simulink model "Vehicle_Model"  (R2018b)
settings: Solver=VariableStepAuto  StartTime=0.0  StopTime=60  FixedStep=0.00000000000000000000000000000000000000001  RelTol=1e-3
undefined symbols (not defined in the file or in its folder): Chassis8_Initial, Initial
(part 2 of 3)

== matlab function Vehicle_Model/MATLAB Function ==
  data: Z output; z input; m_C input; m_WFR input; m_WFL input; m_WRR input; m_WRL input; I_Cy input; I_CFx input; I_CRx input; a input; b input; d_F input; e_F input; d_R input; e_R input; k_SFR input; k_SFL input; k_SRR input; k_SRL input; k_TFR input; k_TFL input; k_TRR input; k_TRL input; c_SFR input; c_SFL input; c_SRR input; c_SRL input; c_TFR input; c_TFL input; c_TRR input; c_TRL input; k_C input; c_C input; F_z input; M_y input; M_xF input; M_xR input; y_FR input; y_FL input; y_RR input; y_RL input; ydot_FR input; ydot_FL input; ydot_RR input; ydot_RL input
function Z = Chassis8(z,m_C,m_WFR,m_WFL,m_WRR,m_WRL,...
    I_Cy,I_CFx,I_CRx,a,b,d_F,e_F,d_R,e_R,k_SFR,k_SFL,k_SRR,k_SRL,...
    k_TFR,k_TFL,k_TRR,k_TRL,c_SFR,c_SFL,c_SRR,c_SRL,c_TFR,c_TFL,...
    c_TRR,c_TRL,k_C,c_C,F_z,M_y,M_xF,M_xR,y_FR,y_FL,y_RR,y_RL,...
    ydot_FR,ydot_FL,ydot_RR,ydot_RL)

Z = [z(2);...
    ...
    (1/m_C) * (F_z...
    + k_SRR * (z(9) - z(1) - b * z(3) + e_R * z(7))...
    + k_SFR * (z(11) - z(1) + a * z(3) + e_F * z(5))...
    + k_SFL * (z(13) - z(1) + a * z(3) - d_F * z(5))...
    + k_SRL * (z(15) - z(1) - b * z(3) - d_R * z(7))...
    + c_SRR * (z(10) - z(2) - b * z(4) + e_R * z(8))...
    + c_SFR * (z(12) - z(2) + a * z(4) + e_F * z(6))...
    + c_SFL * (z(14) - z(2) + a * z(4) - d_F * z(6))...
    + c_SRL * (z(16) - z(2) - b * z(4) - d_R * z(8)));...
    ...
    z(4);...
    ...
    (1/I_Cy) * (M_y...
    + b * k_SRR * (z(9) - z(1) - b * z(3) + e_R * z(7))...
    - a * k_SFR * (z(11) - z(1) + a * z(3) + e_F * z(5))...
    - a * k_SFL * (z(13) - z(1) + a * z(3) - d_F * z(5))...
    + b * k_SRL * (z(15) - z(1) - b * z(3) - d_R * z(7))...
    + b * c_SRR * (z(10) - z(2) - b * z(4) + e_R * z(8))...
    - a * c_SFR * (z(12) - z(2) + a * z(4) + e_F * z(6))...
    - a * c_SFL * (z(14) - z(2) + a * z(4) - d_F * z(6))...
    + b * c_SRL * (z(16) - z(2) - b * z(4) - d_R * z(8)));...
    ...
    z(6);...
    ...
    (1/I_CFx) * (M_xF...
    - e_F * k_SFR * (z(11) - z(1) + a * z(3) + e_F * z(5))...
    + d_F * k_SFL * (z(13) - z(1) + a * z(3) - d_F * z(5))...
    - k_C * (z(5) - z(7))...
    - e_F * c_SFR * (z(12) - z(2) + a * z(4) + e_F * z(6))...
    + d_F * c_SFL * (z(14) - z(2) + a * z(4) - d_F * z(6))...
    - c_C * (z(6) - z(8)));...
    ...
    z(8);...
    ...
    (1/I_CRx) * (M_xR...
    - e_R * k_SRR * (z(9) - z(1) - b * z(3) + e_R * z(7))...
    + d_F * k_SRL * (z(15) - z(1) - b * z(3) - d_R * z(7))...
    + k_C * (z(5) - z(7))...
    - e_R * c_SRR * (z(10) - z(2) - b * z(4) + e_R * z(8))...
    + d_F * c_SRL * (z(16) - z(2) - b * z(4) - d_R * z(8))...
    + c_C * (z(6) - z(8)));...
    ...
    z(10);...
    ...
    (1/m_WRR) * (0 ...
    + k_TRR * (y_RR - z(9))...
    - k_SRR * (z(9) - z(1) - b * z(3) + e_R * z(7))...
    + c_TRR * (ydot_RR - z(10))...
    - c_SRR * (z(10) - z(2) - b * z(4) + e_R * z(8)));...
    ...
    z(12);...
    ...
    (1/m_WFR) * (0 ...
    + k_TFR * (y_FR - z(11))...
    - k_SFR * (z(11) - z(1) + a * z(3) + e_F * z(5))...
    + c_TFR * (ydot_FR - z(12))...
    - c_SFR * (z(12) - z(2) + a * z(4) + e_F * z(6)));...
    ...
    z(14);...
    ...
    (1/m_WFL) * (0 ...
    + k_TFL * (y_FL - z(13))...
    - k_SFL * (z(13) - z(1) + a * z(3) - d_F * z(5))...
    + c_TFL * (ydot_FL - z(14))...
    - c_SFL * (z(14) - z(2) + a * z(4) - d_F * z(6)));...
    ...
    z(16);...
    ...
    (1/m_WRL) * (0 ...
    + k_TRL * (y_RL - z(15))...
    - k_SRL * (z(15) - z(1) - b * z(3) - d_R * z(7))...
    + c_TRL * (ydot_RL - z(16))...
    - c_SRL * (z(16) - z(2) - b * z(4) - d_R * z(8)))...
    ];

end

== matlab function Vehicle_Model/MATLAB Function2 ==
  data: F_z output; M_y output; M_xF output; M_xR output
function [F_z,M_y,M_xF,M_xR] = Forces

% Forces & Moments
g = 9.81;
F_z = -500; %-m_C * g;
M_y = 10;
M_xF = 5;
M_xR = -5;

== matlab function Vehicle_Model/MATLAB Function3 ==
  data: y_FR output; y_FL output; y_RR output; y_RL output
function [y_FR,y_FL,y_RR,y_RL] = Floor_Disp
% Floor Displacements & Velocities
y_FR = 0;
y_FL = 0;
y_RR = 0;
y_RL = 0;

== matlab function Vehicle_Model/MATLAB Function4 ==
  data: k input; F_z output; c input; x input; xdot input
function F_z = Tyre_Force(k,c,x,xdot)

F_z = k * x + c * xdot;

== matlab function Vehicle_Model/MATLAB Function5 ==
  data: k input; F_z output; c input; x input; xdot input
function F_z = Tyre_Force(k,c,x,xdot)

F_z = k * x + c * xdot;

== matlab function Vehicle_Model/MATLAB Function6 ==
  data: k input; F_z output; c input; x input; xdot input
function F_z = Tyre_Force(k,c,x,xdot)

F_z = k * x + c * xdot;

== matlab function Vehicle_Model/MATLAB Function7 ==
  data: k input; F_z output; c input; x input; xdot input
function F_z = Tyre_Force(k,c,x,xdot)

F_z = k * x + c * xdot;

== matlab function Vehicle_Model/MATLAB Function8 ==
  data: Fz input; Fxo output; kappa input; alpha input; gam input; Fzo input; Ro input; q_Bz1 input; q_Bz2 input; q_Bz3 input; q_Bz4 input; q_Bz5 input; q_Bz9 input; q_Bz10 input; q_Cz1 input; q_Dz1 input; q_Dz2 input; q_Dz3 input; q_Dz4 input; q_Dz6 input; q_Dz7 input; q_Dz8 input; q_Dz9 input; q_Ez1 input; q_Ez2 input; q_Ez3 input; q_Ez4 input; q_Ez5 input; q_Hz1 input; q_Hz2 input; q_Hz3 input; q_Hz4 input; p_Cy1 input; p_Dy1 input; p_Dy2 input; p_Dy3 input; p_Ey1 input; p_Ey2 input; p_Ey3 input; p_Ey4 input; p_Ky1 input; p_Ky2 input; p_Ky3 input; p_Hy1 input; p_Hy2 input; p_Hy3 input; p_Vy1 input; p_Vy2 input; p_Vy3 input; p_Vy4 input; p_Cx1 input; p_Dx1 input; p_Dx2 input; p_Ex1 input; p_Ex2 input; p_Ex3 input; p_Ex4 input; p_Kx1 input; p_Kx2 input; p_Kx3 input; p_Hx1 input; p_Hx2 input; p_Vx1 input; p_Vx2 input; car_mu_scaling input; run_info input; Fyo output; Mzo output
function [Fxo,Fyo,Mzo] = Pacejka_Tyre_Model(Fz,kappa,alpha,gam,Fzo,Ro,...
    q_Bz1,q_Bz2,q_Bz3,q_Bz4,q_Bz5,q_Bz9,q_Bz10,q_Cz1,q_Dz1,...
    q_Dz2,q_Dz3,q_Dz4,q_Dz6,q_Dz7,q_Dz8,q_Dz9,q_Ez1,q_Ez2,q_Ez3,q_Ez4,q_Ez5,...
    q_Hz1,q_Hz2,q_Hz3,q_Hz4,p_Cy1,p_Dy1,p_Dy2,p_Dy3,p_Ey1,p_Ey2,p_Ey3,...
    p_Ey4,p_Ky1,p_Ky2,p_Ky3,p_Hy1,p_Hy2,p_Hy3,p_Vy1,p_Vy2,p_Vy3,p_Vy4,...
    p_Cx1,p_Dx1,p_Dx2,p_Ex1,p_Ex2,p_Ex3,p_Ex4,p_Kx1,p_Kx2,p_Kx3,p_Hx1,...
    p_Hx2,p_Vx1,p_Vx2,car_mu_scaling,run_info)
% Pacejka '96 tyre model
%
% Inputs:
% Fz:       normal force (N)
% kappa:    slip ratio (% between -1 and 1) +ve is driving, -ve is braking
% alpha:    slip angle (rad) +ve alpha generates +ve Fyo
% gam:      inclanation angle./camber (rad) +ve indicates top of tyre tipped
%           right
% Outputs:
% Fxo:      Longitudinal force (N)
% Fyo:      Lateral force (N)
% Mzo:      Aligning moment (Nm)


%% tyre coefficients
% each different type of tyre holds different scaling coefficients, load 
% these here. Also loaded are unloaded tyre radius and nominal wheel load

% unpack the structure holding the coefficients
% Get the field names of the structure.
% fields = fieldnames(pacejka_coefs, '-full');
% 
% for ii = 1:length(fields)
%     thisField = fields{ii};
%     create_variable = sprintf('%s = pacejka_coefs.%s;', thisField, thisField);
%     eval(create_variable);
% end
% clear('ii', 'thisField');
% clear('fields', 'create_variable');

%% register track conditions
% scaling factors affected by wet/dry conditions
% if strcmp(run_info.track_conditions,'dry')
    lambda_mux = 1; % peak friction coefficient
    lambda_muy = 1; % peak friction coefficient
% elseif strcmp(run_info.track_conditions,'wet')
%     lambda_mux = 0.5; % peak friction coefficient
%     lambda_muy = 0.5; % peak friction coefficient
% else
%     fprintf('Track conditions incorrectly specified: dry condtitions used \n');
%     lambda_mux = 1; % peak friction coefficient
%     lambda_muy = 1; % peak friction coefficient
% end

% modify with user scaling factor
lambda_mux = lambda_mux*car_mu_scaling;
lambda_muy = lambda_muy*car_mu_scaling;

%% scaling factors
% default values for these values is 1 (except lambda_muV=0)
lambda_Fzo = 1; % nominal rated load
lambda_muV = 0; % with slip speed Vx decaying friction
lambda_Kx = 1; % brake slip stiffness
lambda_Ky = 1; % cornering stiffness
lambda_Cx = 1; % shape factor
lambda_Cy = 1; % shape factor
lambda_Ex = 1; % curvature factor
lambda_Ey = 1; % curvature factor
lambda_Hx = 1; % horizontal shift
lambda_Hy = 1; % horizontal shift
lambda_Vx = 1; % vertical shift
lambda_Vy = 1; % vertical shift
lambda_Kygam = 1; % camber force stiffness
lambda_Kzgam = 1; % camber torque stiffness
lambda_t = 1; % pneumatic trail
lambda_Mr = 1; % residual torque
lambda_ygam = 1;

if ~isrow(kappa) || ~isrow(alpha) || ~isrow(gam)
    kappa = transpose(kappa);
    alpha = transpose(alpha);
    gam = transpose(gam);
end

% for ii=1:length(Fz)
%     %% derived inputs
     dfz = (Fz-Fzo)/Fzo; % normalised change in vertical load
    
    %% longitudinal force (pure longitudinal slip)
    S_Vx = Fz*(p_Vx1+p_Vx2.*dfz).*lambda_Vx.*lambda_mux;
    S_Hx = (p_Hx1+p_Hx2.*dfz).*lambda_Hx;
    kappa_x = kappa + S_Hx;
    K_xk = Fz*(p_Kx1+p_Kx2.*dfz).*exp(-p_Kx3.*dfz).*lambda_Kx;
    E_x = (p_Ex1+p_Ex2.*dfz+p_Ex3.*dfz.^2).*(1-p_Ex4.*sign(kappa_x)).*lambda_Ex;
    mu_x = (p_Dx1+p_Dx2.*dfz).*lambda_mux;
    D_x = mu_x.*Fz;
    C_x = p_Cx1.*lambda_Cx;
    B_x = K_xk./(C_x.*D_x);
    Fxo = D_x.*sin(C_x.*atan(B_x.*kappa_x - E_x.*(B_x.*kappa_x-atan(B_x.*kappa_x)))) + S_Vx;
    
    %% lateral force (pure lateral slip)
    gam_y = gam.*lambda_ygam;
    C_y = p_Cy1.*lambda_Cy;
    mu_y = (p_Dy1+p_Dy2.*dfz).*(1-p_Dy3.*gam.^2).*lambda_muy;
    D_y = mu_y.*Fz;
    S_Hy = (p_Hy1+p_Hy2.*dfz+p_Hy3.*gam).*lambda_Hy;
    alpha_y = alpha + S_Hy;
    E_y = (p_Ey1+p_Ey2.*dfz).*(1-(p_Ey3+p_Ey4.*gam_y).*sign(alpha_y)).*lambda_Ey;
    K_ya = p_Ky1.*Fzo.*sin(2.*atan(Fz./(p_Ky2.*Fzo.*lambda_Fzo))).*(1-p_Ky3.*abs(gam)).*lambda_Fzo.*lambda_Ky;
    B_y = K_ya./(C_y.*D_y);
    S_Vy = Fz.*((p_Vy1+p_Vy2.*dfz)+(p_Vy3+p_Vy4.*dfz).*gam.*lambda_Vy.*lambda_Kygam);
    Fyo = D_y.*sin(C_y.*atan(B_y.*alpha_y - E_y.*(B_y.*alpha_y-atan(B_y.*alpha_y)))) + S_Vy;
    
    %% aligning torque (pure side slip)
    B_t = (q_Bz1+q_Bz2.*dfz+q_Bz3.*dfz.^2).*(1+q_Bz4.*gam.*q_Bz5.*abs(gam)).*lambda_Ky./lambda_muy;
    C_t = q_Cz1;
    D_t = (q_Dz1+q_Dz2.*dfz).*(1+q_Dz3.*gam+q_Dz4.*gam.^2).*Ro.*lambda_t./Fzo;
    S_Ht = q_Hz1+q_Hz2.*dfz+(q_Hz3+q_Hz4.*dfz).*gam;
    alpha_t = alpha + S_Ht;
    E_t = (q_Ez1+q_Ez2.*dfz+q_Ez3.*dfz.^2).*(1+(q_Ez4+q_Ez5.*gam).*atan(B_t.*C_t.*alpha_t));
    B_r = (q_Bz9.*lambda_Ky./lambda_muy+q_Bz10.*B_y.*C_y);
    D_r = Fz.*((q_Dz6+q_Dz7.*dfz)+(q_Dz8+q_Dz9.*dfz).*gam).*Ro.*lambda_muy.*lambda_Mr;
    S_Hf = S_Hy + S_Vy./K_ya;
    alpha_r = alpha + S_Hf;
    Mzr = D_r.*cos(atan(B_r.*alpha_r)).*cos(alpha);
    t = D_t.*cos(C_t.*atan(B_t.*alpha_t-E_t.*(B_t.*alpha_t-atan(B_t.*alpha_t)))).*cos(alpha);
    Mzo = -t.*Fyo + Mzr;
    
% end

== matlab function Vehicle_Model/MATLAB Function9 ==
  data: Fzo output; Ro output; q_Bz1 output; q_Bz2 output; q_Bz3 output; q_Bz4 output; q_Bz5 output; q_Bz9 output; q_Bz10 output; q_Cz1 output; q_Dz1 output; q_Dz2 output; q_Dz3 output; q_Dz4 output; q_Dz6 output; q_Dz7 output; q_Dz8 output; q_Dz9 output; q_Ez1 output; q_Ez2 output; q_Ez3 output; q_Ez4 output; q_Ez5 output; q_Hz1 output; q_Hz2 output; q_Hz3 output; q_Hz4 output; p_Cy1 output; p_Dy1 output; p_Dy2 output; p_Dy3 output; p_Ey1 output; p_Ey2 output; p_Ey3 output; p_Ey4 output; p_Ky1 output; p_Ky2 output; p_Ky3 output; p_Hy1 output; p_Hy2 output; p_Hy3 output; p_Vy1 output; p_Vy2 output; p_Vy3 output; p_Vy4 output; p_Cx1 output; p_Dx1 output; p_Dx2 output; p_Ex1 output; p_Ex2 output; p_Ex3 output; p_Ex4 output; p_Kx1 output; p_Kx2 output; p_Kx3 output; p_Hx1 output; p_Hx2 output; p_Vx1 output; p_Vx2 output
function [Fzo,Ro,q_Bz1,q_Bz2,q_Bz3,q_Bz4,q_Bz5,q_Bz9,q_Bz10,q_Cz1,q_Dz1,...
    q_Dz2,q_Dz3,q_Dz4,q_Dz6,q_Dz7,q_Dz8,q_Dz9,q_Ez1,q_Ez2,q_Ez3,q_Ez4,q_Ez5,...
    q_Hz1,q_Hz2,q_Hz3,q_Hz4,p_Cy1,p_Dy1,p_Dy2,p_Dy3,p_Ey1,p_Ey2,p_Ey3,...
    p_Ey4,p_Ky1,p_Ky2,p_Ky3,p_Hy1,p_Hy2,p_Hy3,p_Vy1,p_Vy2,p_Vy3,p_Vy4,...
    p_Cx1,p_Dx1,p_Dx2,p_Ex1,p_Ex2,p_Ex3,p_Ex4,p_Kx1,p_Kx2,p_Kx3,p_Hx1,...
    p_Hx2,p_Vx1,p_Vx2] = Hoosier_43131
% pacejka model coefficients provided by Stackpole Engineering Services
% for Hoosier tyre model 43131
% as found in the document 'SES_FSAE_Tiredata_Rev1'
% Specs:
% Size	20.0x6.0-13
% Pressure 12 psi


Fzo = 1114.01; % N
Ro = 0.25400; % m

% [ALIGNING COEFFICIENTS]
q_Bz1 =	7.31661;
q_Bz2 =	-1.88850;
q_Bz3 =	-1.22507;
q_Bz4 =	-8.00843;
q_Bz5 =	8.07362;
q_Bz9 =	0;
q_Bz10 = 0;
q_Cz1 =	1.24284;
q_Dz1 =	0.14936;
q_Dz2 =	-0.03781;
q_Dz3 =	0.64550;
q_Dz4 =	0.05268;
q_Dz6 =	-0.02434;
q_Dz7 =	0.01708;
q_Dz8 =	-1.08356;
q_Dz9 =	-0.40710;
q_Ez1 =	-3.38121;
q_Ez2 =	0.10261;
q_Ez3 =	-0.94450;
q_Ez4 =	0.36774;
q_Ez5 =	3.30689;
q_Hz1 =	-0.00061;
q_Hz2 =	-0.00550;
q_Hz3 =	0.38752;
q_Hz4 =	0.43969;

%  [LATERAL COEFFICIENTS]
p_Cy1 =	1.80000;
p_Dy1 =	2.45700;
p_Dy2 =	-0.59060;
p_Dy3 =	11.58940;
p_Ey1 =	0.97472;
p_Ey2 =	0.04076;
p_Ey3 =	0.11095;
p_Ey4 =	-1.20038;
p_Ky1 =	-37.72991;
p_Ky2 =	-1.22482;
p_Ky3 =	1.90662;
p_Hy1 =	0.00081;
p_Hy2 =	-0.00938;
p_Hy3 =	-0.12520;
p_Vy1 =	-0.01307;
p_Vy2 =	0.00121;
p_Vy3 =	-0.21872;
p_Vy4 =	1.77405;

% [LONGITUDINAL COEFFICIENTS]
p_Cx1 =  1.50000;
p_Dx1 =	2.22960;
p_Dx2 =	-0.26506;
p_Ex1 =	0.34731;
p_Ex2 =	-0.36673;
p_Ex3 =	-0.28130;
p_Ex4 =	-0.05543;
p_Kx1 =	46.06520;
p_Kx2 =	-29.43060;
p_Kx3 =	-0.45644;
p_Hx1 =	-0.00087;
p_Hx2 =	-0.00179;
p_Vx1 =	0.00295;
p_Vx2 =	-0.04174;


% export coefficients in structure for ease of passing between functions
% varList = who;
% initialiste oup_ut structure
% pacejka_coefs = struct;

% add all existing variables to struture
% for index = 1:numel(varList)
%     pacejka_coefs.(varList{index}) = eval(varList{index});
% end

== matlab function Vehicle_Model/MATLAB Function10 ==
  data: Fz input; Fxo output; kappa input; alpha input; gam input; Fzo input; Ro input; q_Bz1 input; q_Bz2 input; q_Bz3 input; q_Bz4 input; q_Bz5 input; q_Bz9 input; q_Bz10 input; q_Cz1 input; q_Dz1 input; q_Dz2 input; q_Dz3 input; q_Dz4 input; q_Dz6 input; q_Dz7 input; q_Dz8 input; q_Dz9 input; q_Ez1 input; q_Ez2 input; q_Ez3 input; q_Ez4 input; q_Ez5 input; q_Hz1 input; q_Hz2 input; q_Hz3 input; q_Hz4 input; p_Cy1 input; p_Dy1 input; p_Dy2 input; p_Dy3 input; p_Ey1 input; p_Ey2 input; p_Ey3 input; p_Ey4 input; p_Ky1 input; p_Ky2 input; p_Ky3 input; p_Hy1 input; p_Hy2 input; p_Hy3 input; p_Vy1 input; p_Vy2 input; p_Vy3 input; p_Vy4 input; p_Cx1 input; p_Dx1 input; p_Dx2 input; p_Ex1 input; p_Ex2 input; p_Ex3 input; p_Ex4 input; p_Kx1 input; p_Kx2 input; p_Kx3 input; p_Hx1 input; p_Hx2 input; p_Vx1 input; p_Vx2 input; car_mu_scaling input; run_info input; Fyo output; Mzo output
function [Fxo,Fyo,Mzo] = Pacejka_Tyre_Model(Fz,kappa,alpha,gam,Fzo,Ro,...
    q_Bz1,q_Bz2,q_Bz3,q_Bz4,q_Bz5,q_Bz9,q_Bz10,q_Cz1,q_Dz1,...
    q_Dz2,q_Dz3,q_Dz4,q_Dz6,q_Dz7,q_Dz8,q_Dz9,q_Ez1,q_Ez2,q_Ez3,q_Ez4,q_Ez5,...
    q_Hz1,q_Hz2,q_Hz3,q_Hz4,p_Cy1,p_Dy1,p_Dy2,p_Dy3,p_Ey1,p_Ey2,p_Ey3,...
    p_Ey4,p_Ky1,p_Ky2,p_Ky3,p_Hy1,p_Hy2,p_Hy3,p_Vy1,p_Vy2,p_Vy3,p_Vy4,...
    p_Cx1,p_Dx1,p_Dx2,p_Ex1,p_Ex2,p_Ex3,p_Ex4,p_Kx1,p_Kx2,p_Kx3,p_Hx1,...
    p_Hx2,p_Vx1,p_Vx2,car_mu_scaling,run_info)
% Pacejka '96 tyre model
%
% Inputs:
% Fz:       normal force (N)
% kappa:    slip ratio (% between -1 and 1) +ve is driving, -ve is braking
% alpha:    slip angle (rad) +ve alpha generates +ve Fyo
% gam:      inclanation angle./camber (rad) +ve indicates top of tyre tipped
%           right
% Outputs:
% Fxo:      Longitudinal force (N)
% Fyo:      Lateral force (N)
% Mzo:      Aligning moment (Nm)


%% tyre coefficients
% each different type of tyre holds different scaling coefficients, load 
% these here. Also loaded are unloaded tyre radius and nominal wheel load

% unpack the structure holding the coefficients
% Get the field names of the structure.
% fields = fieldnames(pacejka_coefs, '-full');
% 
% for ii = 1:length(fields)
%     thisField = fields{ii};
%     create_variable = sprintf('%s = pacejka_coefs.%s;', thisField, thisField);
%     eval(create_variable);
% end
% clear('ii', 'thisField');
% clear('fields', 'create_variable');

%% register track conditions
% scaling factors affected by wet/dry conditions
% if strcmp(run_info.track_conditions,'dry')
    lambda_mux = 1; % peak friction coefficient
    lambda_muy = 1; % peak friction coefficient
% elseif strcmp(run_info.track_conditions,'wet')
%     lambda_mux = 0.5; % peak friction coefficient
%     lambda_muy = 0.5; % peak friction coefficient
% else
%     fprintf('Track conditions incorrectly specified: dry condtitions used \n');
%     lambda_mux = 1; % peak friction coefficient
%     lambda_muy = 1; % peak friction coefficient
% end

% modify with user scaling factor
lambda_mux = lambda_mux*car_mu_scaling;
lambda_muy = lambda_muy*car_mu_scaling;

%% scaling factors
% default values for these values is 1 (except lambda_muV=0)
lambda_Fzo = 1; % nominal rated load
lambda_muV = 0; % with slip speed Vx decaying friction
lambda_Kx = 1; % brake slip stiffness
lambda_Ky = 1; % cornering stiffness
lambda_Cx = 1; % shape factor
lambda_Cy = 1; % shape factor
lambda_Ex = 1; % curvature factor
lambda_Ey = 1; % curvature factor
lambda_Hx = 1; % horizontal shift
lambda_Hy = 1; % horizontal shift
lambda_Vx = 1; % vertical shift
lambda_Vy = 1; % vertical shift
lambda_Kygam = 1; % camber force stiffness
lambda_Kzgam = 1; % camber torque stiffness
lambda_t = 1; % pneumatic trail
lambda_Mr = 1; % residual torque
lambda_ygam = 1;

if ~isrow(kappa) || ~isrow(alpha) || ~isrow(gam)
    kappa = transpose(kappa);
    alpha = transpose(alpha);
    gam = transpose(gam);
end

% for ii=1:length(Fz)
%     %% derived inputs
     dfz = (Fz-Fzo)/Fzo; % normalised change in vertical load
    
    %% longitudinal force (pure longitudinal slip)
    S_Vx = Fz*(p_Vx1+p_Vx2.*dfz).*lambda_Vx.*lambda_mux;
    S_Hx = (p_Hx1+p_Hx2.*dfz).*lambda_Hx;
    kappa_x = kappa + S_Hx;
    K_xk = Fz*(p_Kx1+p_Kx2.*dfz).*exp(-p_Kx3.*dfz).*lambda_Kx;
    E_x = (p_Ex1+p_Ex2.*dfz+p_Ex3.*dfz.^2).*(1-p_Ex4.*sign(kappa_x)).*lambda_Ex;
    mu_x = (p_Dx1+p_Dx2.*dfz).*lambda_mux;
    D_x = mu_x.*Fz;
    C_x = p_Cx1.*lambda_Cx;
    B_x = K_xk./(C_x.*D_x);
    Fxo = D_x.*sin(C_x.*atan(B_x.*kappa_x - E_x.*(B_x.*kappa_x-atan(B_x.*kappa_x)))) + S_Vx;
    
    %% lateral force (pure lateral slip)
    gam_y = gam.*lambda_ygam;
    C_y = p_Cy1.*lambda_Cy;
    mu_y = (p_Dy1+p_Dy2.*dfz).*(1-p_Dy3.*gam.^2).*lambda_muy;
    D_y = mu_y.*Fz;
    S_Hy = (p_Hy1+p_Hy2.*dfz+p_Hy3.*gam).*lambda_Hy;
    alpha_y = alpha + S_Hy;
    E_y = (p_Ey1+p_Ey2.*dfz).*(1-(p_Ey3+p_Ey4.*gam_y).*sign(alpha_y)).*lambda_Ey;
    K_ya = p_Ky1.*Fzo.*sin(2.*atan(Fz./(p_Ky2.*Fzo.*lambda_Fzo))).*(1-p_Ky3.*abs(gam)).*lambda_Fzo.*lambda_Ky;
    B_y = K_ya./(C_y.*D_y);
    S_Vy = Fz.*((p_Vy1+p_Vy2.*dfz)+(p_Vy3+p_Vy4.*dfz).*gam.*lambda_Vy.*lambda_Kygam);
    Fyo = D_y.*sin(C_y.*atan(B_y.*alpha_y - E_y.*(B_y.*alpha_y-atan(B_y.*alpha_y)))) + S_Vy;
    
    %% aligning torque (pure side slip)
    B_t = (q_Bz1+q_Bz2.*dfz+q_Bz3.*dfz.^2).*(1+q_Bz4.*gam.*q_Bz5.*abs(gam)).*lambda_Ky./lambda_muy;
    C_t = q_Cz1;
    D_t = (q_Dz1+q_Dz2.*dfz).*(1+q_Dz3.*gam+q_Dz4.*gam.^2).*Ro.*lambda_t./Fzo;
    S_Ht = q_Hz1+q_Hz2.*dfz+(q_Hz3+q_Hz4.*dfz).*gam;
    alpha_t = alpha + S_Ht;
    E_t = (q_Ez1+q_Ez2.*dfz+q_Ez3.*dfz.^2).*(1+(q_Ez4+q_Ez5.*gam).*atan(B_t.*C_t.*alpha_t));
    B_r = (q_Bz9.*lambda_Ky./lambda_muy+q_Bz10.*B_y.*C_y);
    D_r = Fz.*((q_Dz6+q_Dz7.*dfz)+(q_Dz8+q_Dz9.*dfz).*gam).*Ro.*lambda_muy.*lambda_Mr;
    S_Hf = S_Hy + S_Vy./K_ya;
    alpha_r = alpha + S_Hf;
    Mzr = D_r.*cos(atan(B_r.*alpha_r)).*cos(alpha);
    t = D_t.*cos(C_t.*atan(B_t.*alpha_t-E_t.*(B_t.*alpha_t-atan(B_t.*alpha_t)))).*cos(alpha);
    Mzo = -t.*Fyo + Mzr;
    
% end

== matlab function Vehicle_Model/MATLAB Function11 ==
  data: Fzo output; Ro output; q_Bz1 output; q_Bz2 output; q_Bz3 output; q_Bz4 output; q_Bz5 output; q_Bz9 output; q_Bz10 output; q_Cz1 output; q_Dz1 output; q_Dz2 output; q_Dz3 output; q_Dz4 output; q_Dz6 output; q_Dz7 output; q_Dz8 output; q_Dz9 output; q_Ez1 output; q_Ez2 output; q_Ez3 output; q_Ez4 output; q_Ez5 output; q_Hz1 output; q_Hz2 output; q_Hz3 output; q_Hz4 output; p_Cy1 output; p_Dy1 output; p_Dy2 output; p_Dy3 output; p_Ey1 output; p_Ey2 output; p_Ey3 output; p_Ey4 output; p_Ky1 output; p_Ky2 output; p_Ky3 output; p_Hy1 output; p_Hy2 output; p_Hy3 output; p_Vy1 output; p_Vy2 output; p_Vy3 output; p_Vy4 output; p_Cx1 output; p_Dx1 output; p_Dx2 output; p_Ex1 output; p_Ex2 output; p_Ex3 output; p_Ex4 output; p_Kx1 output; p_Kx2 output; p_Kx3 output; p_Hx1 output; p_Hx2 output; p_Vx1 output; p_Vx2 output
function [Fzo,Ro,q_Bz1,q_Bz2,q_Bz3,q_Bz4,q_Bz5,q_Bz9,q_Bz10,q_Cz1,q_Dz1,...
    q_Dz2,q_Dz3,q_Dz4,q_Dz6,q_Dz7,q_Dz8,q_Dz9,q_Ez1,q_Ez2,q_Ez3,q_Ez4,q_Ez5,...
    q_Hz1,q_Hz2,q_Hz3,q_Hz4,p_Cy1,p_Dy1,p_Dy2,p_Dy3,p_Ey1,p_Ey2,p_Ey3,...
    p_Ey4,p_Ky1,p_Ky2,p_Ky3,p_Hy1,p_Hy2,p_Hy3,p_Vy1,p_Vy2,p_Vy3,p_Vy4,...
    p_Cx1,p_Dx1,p_Dx2,p_Ex1,p_Ex2,p_Ex3,p_Ex4,p_Kx1,p_Kx2,p_Kx3,p_Hx1,...
    p_Hx2,p_Vx1,p_Vx2] = Hoosier_43131
% pacejka model coefficients provided by Stackpole Engineering Services
% for Hoosier tyre model 43131
% as found in the document 'SES_FSAE_Tiredata_Rev1'
% Specs:
% Size	20.0x6.0-13
% Pressure 12 psi


Fzo = 1114.01; % N
Ro = 0.25400; % m

% [ALIGNING COEFFICIENTS]
q_Bz1 =	7.31661;
q_Bz2 =	-1.88850;
q_Bz3 =	-1.22507;
q_Bz4 =	-8.00843;
q_Bz5 =	8.07362;
q_Bz9 =	0;
q_Bz10 = 0;
q_Cz1 =	1.24284;
q_Dz1 =	0.14936;
q_Dz2 =	-0.03781;
q_Dz3 =	0.64550;
q_Dz4 =	0.05268;
q_Dz6 =	-0.02434;
q_Dz7 =	0.01708;
q_Dz8 =	-1.08356;
q_Dz9 =	-0.40710;
q_Ez1 =	-3.38121;
q_Ez2 =	0.10261;
q_Ez3 =	-0.94450;
q_Ez4 =	0.36774;
q_Ez5 =	3.30689;
q_Hz1 =	-0.00061;
q_Hz2 =	-0.00550;
q_Hz3 =	0.38752;
q_Hz4 =	0.43969;

%  [LATERAL COEFFICIENTS]
p_Cy1 =	1.80000;
p_Dy1 =	2.45700;
p_Dy2 =	-0.59060;
p_Dy3 =	11.58940;
p_Ey1 =	0.97472;
p_Ey2 =	0.04076;
p_Ey3 =	0.11095;
p_Ey4 =	-1.20038;
p_Ky1 =	-37.72991;
p_Ky2 =	-1.22482;
p_Ky3 =	1.90662;
p_Hy1 =	0.00081;
p_Hy2 =	-0.00938;
p_Hy3 =	-0.12520;
p_Vy1 =	-0.01307;
p_Vy2 =	0.00121;
p_Vy3 =	-0.21872;
p_Vy4 =	1.77405;

% [LONGITUDINAL COEFFICIENTS]
p_Cx1 =  1.50000;
p_Dx1 =	2.22960;
p_Dx2 =	-0.26506;
p_Ex1 =	0.34731;
p_Ex2 =	-0.36673;
p_Ex3 =	-0.28130;
p_Ex4 =	-0.05543;
p_Kx1 =	46.06520;
p_Kx2 =	-29.43060;
p_Kx3 =	-0.45644;
p_Hx1 =	-0.00087;
p_Hx2 =	-0.00179;
p_Vx1 =	0.00295;
p_Vx2 =	-0.04174;


% export coefficients in structure for ease of passing between functions
% varList = who;
% initialiste oup_ut structure
% pacejka_coefs = struct;

% add all existing variables to struture
% for index = 1:numel(varList)
%     pacejka_coefs.(varList{index}) = eval(varList{index});
% end

== matlab function Vehicle_Model/MATLAB Function12 ==
  data: Fz input; Fxo output; kappa input; alpha input; gam input; Fzo input; Ro input; q_Bz1 input; q_Bz2 input; q_Bz3 input; q_Bz4 input; q_Bz5 input; q_Bz9 input; q_Bz10 input; q_Cz1 input; q_Dz1 input; q_Dz2 input; q_Dz3 input; q_Dz4 input; q_Dz6 input; q_Dz7 input; q_Dz8 input; q_Dz9 input; q_Ez1 input; q_Ez2 input; q_Ez3 input; q_Ez4 input; q_Ez5 input; q_Hz1 input; q_Hz2 input; q_Hz3 input; q_Hz4 input; p_Cy1 input; p_Dy1 input; p_Dy2 input; p_Dy3 input; p_Ey1 input; p_Ey2 input; p_Ey3 input; p_Ey4 input; p_Ky1 input; p_Ky2 input; p_Ky3 input; p_Hy1 input; p_Hy2 input; p_Hy3 input; p_Vy1 input; p_Vy2 input; p_Vy3 input; p_Vy4 input; p_Cx1 input; p_Dx1 input; p_Dx2 input; p_Ex1 input; p_Ex2 input; p_Ex3 input; p_Ex4 input; p_Kx1 input; p_Kx2 input; p_Kx3 input; p_Hx1 input; p_Hx2 input; p_Vx1 input; p_Vx2 input; car_mu_scaling input; run_info input; Fyo output; Mzo output
function [Fxo,Fyo,Mzo] = Pacejka_Tyre_Model(Fz,kappa,alpha,gam,Fzo,Ro,...
    q_Bz1,q_Bz2,q_Bz3,q_Bz4,q_Bz5,q_Bz9,q_Bz10,q_Cz1,q_Dz1,...
    q_Dz2,q_Dz3,q_Dz4,q_Dz6,q_Dz7,q_Dz8,q_Dz9,q_Ez1,q_Ez2,q_Ez3,q_Ez4,q_Ez5,...
    q_Hz1,q_Hz2,q_Hz3,q_Hz4,p_Cy1,p_Dy1,p_Dy2,p_Dy3,p_Ey1,p_Ey2,p_Ey3,...
    p_Ey4,p_Ky1,p_Ky2,p_Ky3,p_Hy1,p_Hy2,p_Hy3,p_Vy1,p_Vy2,p_Vy3,p_Vy4,...
    p_Cx1,p_Dx1,p_Dx2,p_Ex1,p_Ex2,p_Ex3,p_Ex4,p_Kx1,p_Kx2,p_Kx3,p_Hx1,...
    p_Hx2,p_Vx1,p_Vx2,car_mu_scaling,run_info)
% Pacejka '96 tyre model
%
% Inputs:
% Fz:       normal force (N)
% kappa:    slip ratio (% between -1 and 1) +ve is driving, -ve is braking
% alpha:    slip angle (rad) +ve alpha generates +ve Fyo
% gam:      inclanation angle./camber (rad) +ve indicates top of tyre tipped
%           right
% Outputs:
% Fxo:      Longitudinal force (N)
% Fyo:      Lateral force (N)
% Mzo:      Aligning moment (Nm)


%% tyre coefficients
% each different type of tyre holds different scaling coefficients, load 
% these here. Also loaded are unloaded tyre radius and nominal wheel load

% unpack the structure holding the coefficients
% Get the field names of the structure.
% fields = fieldnames(pacejka_coefs, '-full');
% 
% for ii = 1:length(fields)
%     thisField = fields{ii};
%     create_variable = sprintf('%s = pacejka_coefs.%s;', thisField, thisField);
%     eval(create_variable);
% end
% clear('ii', 'thisField');
% clear('fields', 'create_variable');

%% register track conditions
% scaling factors affected by wet/dry conditions
% if strcmp(run_info.track_conditions,'dry')
    lambda_mux = 1; % peak friction coefficient
    lambda_muy = 1; % peak friction coefficient
% elseif strcmp(run_info.track_conditions,'wet')
%     lambda_mux = 0.5; % peak friction coefficient
%     lambda_muy = 0.5; % peak friction coefficient
% else
%     fprintf('Track conditions incorrectly specified: dry condtitions used \n');
%     lambda_mux = 1; % peak friction coefficient
%     lambda_muy = 1; % peak friction coefficient
% end

% modify with user scaling factor
lambda_mux = lambda_mux*car_mu_scaling;
lambda_muy = lambda_muy*car_mu_scaling;

%% scaling factors
% default values for these values is 1 (except lambda_muV=0)
lambda_Fzo = 1; % nominal rated load
lambda_muV = 0; % with slip speed Vx decaying friction
lambda_Kx = 1; % brake slip stiffness
lambda_Ky = 1; % cornering stiffness
lambda_Cx = 1; % shape factor
lambda_Cy = 1; % shape factor
lambda_Ex = 1; % curvature factor
lambda_Ey = 1; % curvature factor
lambda_Hx = 1; % horizontal shift
lambda_Hy = 1; % horizontal shift
lambda_Vx = 1; % vertical shift
lambda_Vy = 1; % vertical shift
lambda_Kygam = 1; % camber force stiffness
lambda_Kzgam = 1; % camber torque stiffness
lambda_t = 1; % pneumatic trail
lambda_Mr = 1; % residual torque
lambda_ygam = 1;

if ~isrow(kappa) || ~isrow(alpha) || ~isrow(gam)
    kappa = transpose(kappa);
    alpha = transpose(alpha);
    gam = transpose(gam);
end

% for ii=1:length(Fz)
%     %% derived inputs
     dfz = (Fz-Fzo)/Fzo; % normalised change in vertical load
    
    %% longitudinal force (pure longitudinal slip)
    S_Vx = Fz*(p_Vx1+p_Vx2.*dfz).*lambda_Vx.*lambda_mux;
    S_Hx = (p_Hx1+p_Hx2.*dfz).*lambda_Hx;
    kappa_x = kappa + S_Hx;
    K_xk = Fz*(p_Kx1+p_Kx2.*dfz).*exp(-p_Kx3.*dfz).*lambda_Kx;
    E_x = (p_Ex1+p_Ex2.*dfz+p_Ex3.*dfz.^2).*(1-p_Ex4.*sign(kappa_x)).*lambda_Ex;
    mu_x = (p_Dx1+p_Dx2.*dfz).*lambda_mux;
    D_x = mu_x.*Fz;
    C_x = p_Cx1.*lambda_Cx;
    B_x = K_xk./(C_x.*D_x);
    Fxo = D_x.*sin(C_x.*atan(B_x.*kappa_x - E_x.*(B_x.*kappa_x-atan(B_x.*kappa_x)))) + S_Vx;
    
    %% lateral force (pure lateral slip)
    gam_y = gam.*lambda_ygam;
    C_y = p_Cy1.*lambda_Cy;
    mu_y = (p_Dy1+p_Dy2.*dfz).*(1-p_Dy3.*gam.^2).*lambda_muy;
    D_y = mu_y.*Fz;
    S_Hy = (p_Hy1+p_Hy2.*dfz+p_Hy3.*gam).*lambda_Hy;
    alpha_y = alpha + S_Hy;
    E_y = (p_Ey1+p_Ey2.*dfz).*(1-(p_Ey3+p_Ey4.*gam_y).*sign(alpha_y)).*lambda_Ey;
    K_ya = p_Ky1.*Fzo.*sin(2.*atan(Fz./(p_Ky2.*Fzo.*lambda_Fzo))).*(1-p_Ky3.*abs(gam)).*lambda_Fzo.*lambda_Ky;
    B_y = K_ya./(C_y.*D_y);
    S_Vy = Fz.*((p_Vy1+p_Vy2.*dfz)+(p_Vy3+p_Vy4.*dfz).*gam.*lambda_Vy.*lambda_Kygam);
    Fyo = D_y.*sin(C_y.*atan(B_y.*alpha_y - E_y.*(B_y.*alpha_y-atan(B_y.*alpha_y)))) + S_Vy;
    
    %% aligning torque (pure side slip)
    B_t = (q_Bz1+q_Bz2.*dfz+q_Bz3.*dfz.^2).*(1+q_Bz4.*gam.*q_Bz5.*abs(gam)).*lambda_Ky./lambda_muy;
    C_t = q_Cz1;
    D_t = (q_Dz1+q_Dz2.*dfz).*(1+q_Dz3.*gam+q_Dz4.*gam.^2).*Ro.*lambda_t./Fzo;
    S_Ht = q_Hz1+q_Hz2.*dfz+(q_Hz3+q_Hz4.*dfz).*gam;
    alpha_t = alpha + S_Ht;
    E_t = (q_Ez1+q_Ez2.*dfz+q_Ez3.*dfz.^2).*(1+(q_Ez4+q_Ez5.*gam).*atan(B_t.*C_t.*alpha_t));
    B_r = (q_Bz9.*lambda_Ky./lambda_muy+q_Bz10.*B_y.*C_y);
    D_r = Fz.*((q_Dz6+q_Dz7.*dfz)+(q_Dz8+q_Dz9.*dfz).*gam).*Ro.*lambda_muy.*lambda_Mr;
    S_Hf = S_Hy + S_Vy./K_ya;
    alpha_r = alpha + S_Hf;
    Mzr = D_r.*cos(atan(B_r.*alpha_r)).*cos(alpha);
    t = D_t.*cos(C_t.*atan(B_t.*alpha_t-E_t.*(B_t.*alpha_t-atan(B_t.*alpha_t)))).*cos(alpha);
    Mzo = -t.*Fyo + Mzr;
    
% end

== matlab function Vehicle_Model/MATLAB Function13 ==
  data: Fzo output; Ro output; q_Bz1 output; q_Bz2 output; q_Bz3 output; q_Bz4 output; q_Bz5 output; q_Bz9 output; q_Bz10 output; q_Cz1 output; q_Dz1 output; q_Dz2 output; q_Dz3 output; q_Dz4 output; q_Dz6 output; q_Dz7 output; q_Dz8 output; q_Dz9 output; q_Ez1 output; q_Ez2 output; q_Ez3 output; q_Ez4 output; q_Ez5 output; q_Hz1 output; q_Hz2 output; q_Hz3 output; q_Hz4 output; p_Cy1 output; p_Dy1 output; p_Dy2 output; p_Dy3 output; p_Ey1 output; p_Ey2 output; p_Ey3 output; p_Ey4 output; p_Ky1 output; p_Ky2 output; p_Ky3 output; p_Hy1 output; p_Hy2 output; p_Hy3 output; p_Vy1 output; p_Vy2 output; p_Vy3 output; p_Vy4 output; p_Cx1 output; p_Dx1 output; p_Dx2 output; p_Ex1 output; p_Ex2 output; p_Ex3 output; p_Ex4 output; p_Kx1 output; p_Kx2 output; p_Kx3 output; p_Hx1 output; p_Hx2 output; p_Vx1 output; p_Vx2 output
function [Fzo,Ro,q_Bz1,q_Bz2,q_Bz3,q_Bz4,q_Bz5,q_Bz9,q_Bz10,q_Cz1,q_Dz1,...
    q_Dz2,q_Dz3,q_Dz4,q_Dz6,q_Dz7,q_Dz8,q_Dz9,q_Ez1,q_Ez2,q_Ez3,q_Ez4,q_Ez5,...
    q_Hz1,q_Hz2,q_Hz3,q_Hz4,p_Cy1,p_Dy1,p_Dy2,p_Dy3,p_Ey1,p_Ey2,p_Ey3,...
    p_Ey4,p_Ky1,p_Ky2,p_Ky3,p_Hy1,p_Hy2,p_Hy3,p_Vy1,p_Vy2,p_Vy3,p_Vy4,...
    p_Cx1,p_Dx1,p_Dx2,p_Ex1,p_Ex2,p_Ex3,p_Ex4,p_Kx1,p_Kx2,p_Kx3,p_Hx1,...
    p_Hx2,p_Vx1,p_Vx2] = Hoosier_43131
% pacejka model coefficients provided by Stackpole Engineering Services
% for Hoosier tyre model 43131
% as found in the document 'SES_FSAE_Tiredata_Rev1'
% Specs:
% Size	20.0x6.0-13
% Pressure 12 psi


Fzo = 1114.01; % N
Ro = 0.25400; % m

% [ALIGNING COEFFICIENTS]
q_Bz1 =	7.31661;
q_Bz2 =	-1.88850;
q_Bz3 =	-1.22507;
q_Bz4 =	-8.00843;
q_Bz5 =	8.07362;
q_Bz9 =	0;
q_Bz10 = 0;
q_Cz1 =	1.24284;
q_Dz1 =	0.14936;
q_Dz2 =	-0.03781;
q_Dz3 =	0.64550;
q_Dz4 =	0.05268;
q_Dz6 =	-0.02434;
q_Dz7 =	0.01708;
q_Dz8 =	-1.08356;
q_Dz9 =	-0.40710;
q_Ez1 =	-3.38121;
q_Ez2 =	0.10261;
q_Ez3 =	-0.94450;
q_Ez4 =	0.36774;
q_Ez5 =	3.30689;
q_Hz1 =	-0.00061;
q_Hz2 =	-0.00550;
q_Hz3 =	0.38752;
q_Hz4 =	0.43969;

%  [LATERAL COEFFICIENTS]
p_Cy1 =	1.80000;
p_Dy1 =	2.45700;
p_Dy2 =	-0.59060;
p_Dy3 =	11.58940;
p_Ey1 =	0.97472;
p_Ey2 =	0.04076;
p_Ey3 =	0.11095;
p_Ey4 =	-1.20038;
p_Ky1 =	-37.72991;
p_Ky2 =	-1.22482;
p_Ky3 =	1.90662;
p_Hy1 =	0.00081;
p_Hy2 =	-0.00938;
p_Hy3 =	-0.12520;
p_Vy1 =	-0.01307;
p_Vy2 =	0.00121;
p_Vy3 =	-0.21872;
p_Vy4 =	1.77405;

% [LONGITUDINAL COEFFICIENTS]
p_Cx1 =  1.50000;
p_Dx1 =	2.22960;
p_Dx2 =	-0.26506;
p_Ex1 =	0.34731;
p_Ex2 =	-0.36673;
p_Ex3 =	-0.28130;
p_Ex4 =	-0.05543;
p_Kx1 =	46.06520;
p_Kx2 =	-29.43060;
p_Kx3 =	-0.45644;
p_Hx1 =	-0.00087;
p_Hx2 =	-0.00179;
p_Vx1 =	0.00295;
p_Vx2 =	-0.04174;


% export coefficients in structure for ease of passing between functions
% varList = who;
% initialiste oup_ut structure
% pacejka_coefs = struct;

% add all existing variables to struture
% for index = 1:numel(varList)
%     pacejka_coefs.(varList{index}) = eval(varList{index});
% end

== matlab function Vehicle_Model/MATLAB Function14 ==
  data: Fz input; Fxo output; kappa input; alpha input; gam input; Fzo input; Ro input; q_Bz1 input; q_Bz2 input; q_Bz3 input; q_Bz4 input; q_Bz5 input; q_Bz9 input; q_Bz10 input; q_Cz1 input; q_Dz1 input; q_Dz2 input; q_Dz3 input; q_Dz4 input; q_Dz6 input; q_Dz7 input; q_Dz8 input; q_Dz9 input; q_Ez1 input; q_Ez2 input; q_Ez3 input; q_Ez4 input; q_Ez5 input; q_Hz1 input; q_Hz2 input; q_Hz3 input; q_Hz4 input; p_Cy1 input; p_Dy1 input; p_Dy2 input; p_Dy3 input; p_Ey1 input; p_Ey2 input; p_Ey3 input; p_Ey4 input; p_Ky1 input; p_Ky2 input; p_Ky3 input; p_Hy1 input; p_Hy2 input; p_Hy3 input; p_Vy1 input; p_Vy2 input; p_Vy3 input; p_Vy4 input; p_Cx1 input; p_Dx1 input; p_Dx2 input; p_Ex1 input; p_Ex2 input; p_Ex3 input; p_Ex4 input; p_Kx1 input; p_Kx2 input; p_Kx3 input; p_Hx1 input; p_Hx2 input; p_Vx1 input; p_Vx2 input; car_mu_scaling input; run_info input; Fyo output; Mzo output
function [Fxo,Fyo,Mzo] = Pacejka_Tyre_Model(Fz,kappa,alpha,gam,Fzo,Ro,...
    q_Bz1,q_Bz2,q_Bz3,q_Bz4,q_Bz5,q_Bz9,q_Bz10,q_Cz1,q_Dz1,...
    q_Dz2,q_Dz3,q_Dz4,q_Dz6,q_Dz7,q_Dz8,q_Dz9,q_Ez1,q_Ez2,q_Ez3,q_Ez4,q_Ez5,...
    q_Hz1,q_Hz2,q_Hz3,q_Hz4,p_Cy1,p_Dy1,p_Dy2,p_Dy3,p_Ey1,p_Ey2,p_Ey3,...
    p_Ey4,p_Ky1,p_Ky2,p_Ky3,p_Hy1,p_Hy2,p_Hy3,p_Vy1,p_Vy2,p_Vy3,p_Vy4,...
    p_Cx1,p_Dx1,p_Dx2,p_Ex1,p_Ex2,p_Ex3,p_Ex4,p_Kx1,p_Kx2,p_Kx3,p_Hx1,...
    p_Hx2,p_Vx1,p_Vx2,car_mu_scaling,run_info)
% Pacejka '96 tyre model
%
% Inputs:
% Fz:       normal force (N)
% kappa:    slip ratio (% between -1 and 1) +ve is driving, -ve is braking
% alpha:    slip angle (rad) +ve alpha generates +ve Fyo
% gam:      inclanation angle./camber (rad) +ve indicates top of tyre tipped
%           right
% Outputs:
% Fxo:      Longitudinal force (N)
% Fyo:      Lateral force (N)
% Mzo:      Aligning moment (Nm)


%% tyre coefficients
% each different type of tyre holds different scaling coefficients, load 
% these here. Also loaded are unloaded tyre radius and nominal wheel load

% unpack the structure holding the coefficients
% Get the field names of the structure.
% fields = fieldnames(pacejka_coefs, '-full');
% 
% for ii = 1:length(fields)
%     thisField = fields{ii};
%     create_variable = sprintf('%s = pacejka_coefs.%s;', thisField, thisField);
%     eval(create_variable);
% end
% clear('ii', 'thisField');
% clear('fields', 'create_variable');

%% register track conditions
% scaling factors affected by wet/dry conditions
% if strcmp(run_info.track_conditions,'dry')
    lambda_mux = 1; % peak friction coefficient
    lambda_muy = 1; % peak friction coefficient
% elseif strcmp(run_info.track_conditions,'wet')
%     lambda_mux = 0.5; % peak friction coefficient
%     lambda_muy = 0.5; % peak friction coefficient
% else
%     fprintf('Track conditions incorrectly specified: dry condtitions used \n');
%     lambda_mux = 1; % peak friction coefficient
%     lambda_muy = 1; % peak friction coefficient
% end

% modify with user scaling factor
lambda_mux = lambda_mux*car_mu_scaling;
lambda_muy = lambda_muy*car_mu_scaling;

%% scaling factors
% default values for these values is 1 (except lambda_muV=0)
lambda_Fzo = 1; % nominal rated load
lambda_muV = 0; % with slip speed Vx decaying friction
lambda_Kx = 1; % brake slip stiffness
lambda_Ky = 1; % cornering stiffness
lambda_Cx = 1; % shape factor
lambda_Cy = 1; % shape factor
lambda_Ex = 1; % curvature factor
lambda_Ey = 1; % curvature factor
lambda_Hx = 1; % horizontal shift
lambda_Hy = 1; % horizontal shift
lambda_Vx = 1; % vertical shift
lambda_Vy = 1; % vertical shift
lambda_Kygam = 1; % camber force stiffness
lambda_Kzgam = 1; % camber torque stiffness
lambda_t = 1; % pneumatic trail
lambda_Mr = 1; % residual torque
lambda_ygam = 1;

if ~isrow(kappa) || ~isrow(alpha) || ~isrow(gam)
    kappa = transpose(kappa);
    alpha = transpose(alpha);
    gam = transpose(gam);
end

% for ii=1:length(Fz)
%     %% derived inputs
     dfz = (Fz-Fzo)/Fzo; % normalised change in vertical load
    
    %% longitudinal force (pure longitudinal slip)
    S_Vx = Fz*(p_Vx1+p_Vx2.*dfz).*lambda_Vx.*lambda_mux;
    S_Hx = (p_Hx1+p_Hx2.*dfz).*lambda_Hx;
    kappa_x = kappa + S_Hx;
    K_xk = Fz*(p_Kx1+p_Kx2.*dfz).*exp(-p_Kx3.*dfz).*lambda_Kx;
    E_x = (p_Ex1+p_Ex2.*dfz+p_Ex3.*dfz.^2).*(1-p_Ex4.*sign(kappa_x)).*lambda_Ex;
    mu_x = (p_Dx1+p_Dx2.*dfz).*lambda_mux;
    D_x = mu_x.*Fz;
    C_x = p_Cx1.*lambda_Cx;
    B_x = K_xk./(C_x.*D_x);
    Fxo = D_x.*sin(C_x.*atan(B_x.*kappa_x - E_x.*(B_x.*kappa_x-atan(B_x.*kappa_x)))) + S_Vx;
    
    %% lateral force (pure lateral slip)
    gam_y = gam.*lambda_ygam;
    C_y = p_Cy1.*lambda_Cy;
    mu_y = (p_Dy1+p_Dy2.*dfz).*(1-p_Dy3.*gam.^2).*lambda_muy;
    D_y = mu_y.*Fz;
    S_Hy = (p_Hy1+p_Hy2.*dfz+p_Hy3.*gam).*lambda_Hy;
    alpha_y = alpha + S_Hy;
    E_y = (p_Ey1+p_Ey2.*dfz).*(1-(p_Ey3+p_Ey4.*gam_y).*sign(alpha_y)).*lambda_Ey;
    K_ya = p_Ky1.*Fzo.*sin(2.*atan(Fz./(p_Ky2.*Fzo.*lambda_Fzo))).*(1-p_Ky3.*abs(gam)).*lambda_Fzo.*lambda_Ky;
    B_y = K_ya./(C_y.*D_y);
    S_Vy = Fz.*((p_Vy1+p_Vy2.*dfz)+(p_Vy3+p_Vy4.*dfz).*gam.*lambda_Vy.*lambda_Kygam);
    Fyo = D_y.*sin(C_y.*atan(B_y.*alpha_y - E_y.*(B_y.*alpha_y-atan(B_y.*alpha_y)))) + S_Vy;
    
    %% aligning torque (pure side slip)
    B_t = (q_Bz1+q_Bz2.*dfz+q_Bz3.*dfz.^2).*(1+q_Bz4.*gam.*q_Bz5.*abs(gam)).*lambda_Ky./lambda_muy;
    C_t = q_Cz1;
    D_t = (q_Dz1+q_Dz2.*dfz).*(1+q_Dz3.*gam+q_Dz4.*gam.^2).*Ro.*lambda_t./Fzo;
    S_Ht = q_Hz1+q_Hz2.*dfz+(q_Hz3+q_Hz4.*dfz).*gam;
    alpha_t = alpha + S_Ht;
    E_t = (q_Ez1+q_Ez2.*dfz+q_Ez3.*dfz.^2).*(1+(q_Ez4+q_Ez5.*gam).*atan(B_t.*C_t.*alpha_t));
    B_r = (q_Bz9.*lambda_Ky./lambda_muy+q_Bz10.*B_y.*C_y);
    D_r = Fz.*((q_Dz6+q_Dz7.*dfz)+(q_Dz8+q_Dz9.*dfz).*gam).*Ro.*lambda_muy.*lambda_Mr;
    S_Hf = S_Hy + S_Vy./K_ya;
    alpha_r = alpha + S_Hf;
    Mzr = D_r.*cos(atan(B_r.*alpha_r)).*cos(alpha);
    t = D_t.*cos(C_t.*atan(B_t.*alpha_t-E_t.*(B_t.*alpha_t-atan(B_t.*alpha_t)))).*cos(alpha);
    Mzo = -t.*Fyo + Mzr;
    
% end

== matlab function Vehicle_Model/MATLAB Function15 ==
  data: Fzo output; Ro output; q_Bz1 output; q_Bz2 output; q_Bz3 output; q_Bz4 output; q_Bz5 output; q_Bz9 output; q_Bz10 output; q_Cz1 output; q_Dz1 output; q_Dz2 output; q_Dz3 output; q_Dz4 output; q_Dz6 output; q_Dz7 output; q_Dz8 output; q_Dz9 output; q_Ez1 output; q_Ez2 output; q_Ez3 output; q_Ez4 output; q_Ez5 output; q_Hz1 output; q_Hz2 output; q_Hz3 output; q_Hz4 output; p_Cy1 output; p_Dy1 output; p_Dy2 output; p_Dy3 output; p_Ey1 output; p_Ey2 output; p_Ey3 output; p_Ey4 output; p_Ky1 output; p_Ky2 output; p_Ky3 output; p_Hy1 output; p_Hy2 output; p_Hy3 output; p_Vy1 output; p_Vy2 output; p_Vy3 output; p_Vy4 output; p_Cx1 output; p_Dx1 output; p_Dx2 output; p_Ex1 output; p_Ex2 output; p_Ex3 output; p_Ex4 output; p_Kx1 output; p_Kx2 output; p_Kx3 output; p_Hx1 output; p_Hx2 output; p_Vx1 output; p_Vx2 output
function [Fzo,Ro,q_Bz1,q_Bz2,q_Bz3,q_Bz4,q_Bz5,q_Bz9,q_Bz10,q_Cz1,q_Dz1,...
    q_Dz2,q_Dz3,q_Dz4,q_Dz6,q_Dz7,q_Dz8,q_Dz9,q_Ez1,q_Ez2,q_Ez3,q_Ez4,q_Ez5,...
    q_Hz1,q_Hz2,q_Hz3,q_Hz4,p_Cy1,p_Dy1,p_Dy2,p_Dy3,p_Ey1,p_Ey2,p_Ey3,...
    p_Ey4,p_Ky1,p_Ky2,p_Ky3,p_Hy1,p_Hy2,p_Hy3,p_Vy1,p_Vy2,p_Vy3,p_Vy4,...
    p_Cx1,p_Dx1,p_Dx2,p_Ex1,p_Ex2,p_Ex3,p_Ex4,p_Kx1,p_Kx2,p_Kx3,p_Hx1,...
    p_Hx2,p_Vx1,p_Vx2] = Hoosier_43131
% pacejka model coefficients provided by Stackpole Engineering Services
% for Hoosier tyre model 43131
% as found in the document 'SES_FSAE_Tiredata_Rev1'
% Specs:
% Size	20.0x6.0-13
% Pressure 12 psi


Fzo = 1114.01; % N
Ro = 0.25400; % m

% [ALIGNING COEFFICIENTS]
q_Bz1 =	7.31661;
q_Bz2 =	-1.88850;
q_Bz3 =	-1.22507;
q_Bz4 =	-8.00843;
q_Bz5 =	8.07362;
q_Bz9 =	0;
q_Bz10 = 0;
q_Cz1 =	1.24284;
q_Dz1 =	0.14936;
q_Dz2 =	-0.03781;
q_Dz3 =	0.64550;
q_Dz4 =	0.05268;
q_Dz6 =	-0.02434;
q_Dz7 =	0.01708;
q_Dz8 =	-1.08356;
q_Dz9 =	-0.40710;
q_Ez1 =	-3.38121;
q_Ez2 =	0.10261;
q_Ez3 =	-0.94450;
q_Ez4 =	0.36774;
q_Ez5 =	3.30689;
q_Hz1 =	-0.00061;
q_Hz2 =	-0.00550;
q_Hz3 =	0.38752;
q_Hz4 =	0.43969;

%  [LATERAL COEFFICIENTS]
p_Cy1 =	1.80000;
p_Dy1 =	2.45700;
p_Dy2 =	-0.59060;
p_Dy3 =	11.58940;
p_Ey1 =	0.97472;
p_Ey2 =	0.04076;
p_Ey3 =	0.11095;
p_Ey4 =	-1.20038;
p_Ky1 =	-37.72991;
p_Ky2 =	-1.22482;
p_Ky3 =	1.90662;
p_Hy1 =	0.00081;
p_Hy2 =	-0.00938;
p_Hy3 =	-0.12520;
p_Vy1 =	-0.01307;
p_Vy2 =	0.00121;
p_Vy3 =	-0.21872;
p_Vy4 =	1.77405;

% [LONGITUDINAL COEFFICIENTS]
p_Cx1 =  1.50000;
p_Dx1 =	2.22960;
p_Dx2 =	-0.26506;
p_Ex1 =	0.34731;
p_Ex2 =	-0.36673;
p_Ex3 =	-0.28130;
p_Ex4 =	-0.05543;
p_Kx1 =	46.06520;
p_Kx2 =	-29.43060;
p_Kx3 =	-0.45644;
p_Hx1 =	-0.00087;
p_Hx2 =	-0.00179;
p_Vx1 =	0.00295;
p_Vx2 =	-0.04174;


% export coefficients in structure for ease of passing between functions
% varList = who;
% initialiste oup_ut structure
% pacejka_coefs = struct;

% add all existing variables to struture
% for index = 1:numel(varList)
%     pacejka_coefs.(varList{index}) = eval(varList{index});
% end

== matlab function Vehicle_Model/MATLAB Function16 ==
  data: m_C input; v_x output; v_x input; r input; F_y input
function v_x = Brakes(m_C, v_x, r, F_y)

if (m_C*v_x^2)/r - F_y > 0
    v_x = (F_y*r/m_C)^0.5;
end

== matlab function Vehicle_Model/MATLAB Function17 ==
  data: m_C output; m_CF output; m_CR output; m_WFR output; m_WFL output; m_WRR output; m_WRL output; I_Cy output; I_CFx output; I_CRx output; a output; b output; d_F output; e_F output; d_R output; e_R output; k_C output; c_C output; h_C output; h_CF output; h_CR output; mu_scaling output
function [m_C,m_CF,m_CR,m_WFR,m_WFL,m_WRR,m_WRL,I_Cy,I_CFx,I_CRx,a,b,d_F,...
    e_F,d_R,e_R,k_C,c_C,h_C,h_CF,h_CR,mu_scaling] = Car_Parameters
%% Car Parameters
% Masses
m_C = 200; %car sprung mass (kg)
m_CF = 100;
m_CR = m_C - m_CF;
m_WFR = 5; %front right wheel mass (kg)
m_WFL = 5; %front left wheel mass (kg)
m_WRR = 5; %rear right wheel mass (kg)
m_WRL = 5; %rear left wheel mass (kg)

% Intertias
I_Cy = 1000; %chassis interia around y (kg m^2)
I_CFx = 500; %chassis front inertia around x (kg m^2)
I_CRx = 500; %chassis rear inertia around x (kg m^2)

% Geometries
a = 0.8; %distance of COG from front axle (m)
b = 0.8; %distance of COG from rear axle (m)
d_F = 0.6; %distance of COG from front left tire (m)
e_F = 0.6; %distance of COG from front right tire (m)
d_R = 0.6; %distance of COG from rear left tire (m)
e_R = 0.6; %distance of COG from rear right tire (m)
h_C = 0.4;
h_CF = 0.4;
h_CR = 0.4;

% Other Stiffnesses
k_C = 2000;

% Other Damping Coefficients
c_C = 1000;

% mu
mu_scaling = 0.5;

== matlab function Vehicle_Model/MATLAB Function18 ==
  data: g input; F_y output; m_C input; h_C input; m_CF input; m_CR input; h_CF input; h_CR input; a input; b input; d_F input; e_F input; d_R input; e_R input; F_yFR input; F_yFL input; F_yRR input; F_yRL input; F_xFR input; F_xFL input; F_xRR input; F_xRL input; M_zFR input; M_zFL input; M_zRR input; M_zRL input; S_FR input; S_FL input; S_RR input; S_RL input; m_WRL input; m_WRR input; m_WFL input; m_WFR input; F_x output; M_z output; M_y output; M_xF output; M_xR output; F_z output
function [F_y,F_x,M_z,M_y,M_xF,M_xR,F_z] = Chassis7(g,m_C,h_C,m_CF,m_CR,...
    h_CF,h_CR,a,b,d_F,e_F,d_R,e_R,F_yFR,F_yFL,F_yRR,F_yRL,F_xFR,F_xFL,...
    F_xRR,F_xRL,M_zFR,M_zFL,M_zRR,M_zRL,S_FR,S_FL,S_RR,S_RL,m_WRL,m_WRR,...
    m_WFL,m_WFR)

F_y = F_yRL * cos(S_RL) + F_yRR * cos(S_RR) + F_yFL * cos(S_FL) + ...
    F_yFR * cos(S_FR)...
     - F_xRL * sin(S_RL) - F_xRR * sin(S_RR) + F_xFL * sin(S_FL) + ...
    F_xFR * sin(S_FR);

F_x = F_xRL * cos(S_RL) + F_xRR * cos(S_RR) + F_xFL * cos(S_FL) + ...
    F_xFR * cos(S_FR)...
     + F_yRL * sin(S_RL) + F_yRR * sin(S_RR) - F_yFL * sin(S_FL) - ...
    F_yFR * sin(S_FR);

F_z = -g * m_C;

M_z = F_xRR * (sin(S_RR) * b + cos(S_RR) * e_R) +...
    F_yRR * (sin(S_RR) * e_R - cos(S_RR) * b) +...
    F_xFR * (cos(S_FR) * e_F + sin(S_FR) * a) +...
    F_yFR * (cos(S_FR) * a - sin(S_FR) * e_F) +...
    F_xFL * (-cos(S_FL) * d_F + sin(S_FL) * a) +...
    F_yFL * (cos(S_FL) * a + sin(S_FL) * d_F) +...
    F_xRL * (-cos(S_RL) * d_R + sin(S_RL) * b) +...
    F_yRL * (-sin(S_RL) * d_R - cos(S_RL) * b) +...
    + M_zFL + M_zRL + M_zRR + M_zFR;

m = m_C + m_WRL + m_WRR + m_WFL + m_WFR;
a_x = F_x / m;
a_y = F_y / m;
M_y = m_C * a_x * h_C;
M_xF = m_CF * a_y * h_CF;
M_xR = m_CR * a_y * h_CR;

== matlab function Vehicle_Model/MATLAB Function19 ==
  data: y_FR output; y_FL output; y_RR output; y_RL output; t input
function [y_FR,y_FL,y_RR,y_RL] = Floor_Disp(t)
% Floor Displacements & Velocities
y_FR = 0;% 0.01 * sin(t) *exp(-0.1*t);
y_FL = 0;
y_RR = 0;
y_RL = 0;

== matlab function Vehicle_Model/Chassis Vertical 8DOF/MATLAB Function19 ==
  data: Z output; z input; m_C input; m_WFR input; m_WFL input; m_WRR input; m_WRL input; I_Cy input; I_CFx input; I_CRx input; a input; b input; d_F input; e_F input; d_R input; e_R input; k_C input; c_C input; k_SFR input; k_SFL input; k_SRR input; k_SRL input; k_TFR input; k_TFL input; k_TRR input; k_TRL input; c_SFR input; c_SFL input; c_SRR input; c_SRL input; c_TFR input; c_TFL input; c_TRR input; c_TRL input; F_zC input; M_y input; M_xF input; M_xR input; F_zWFR input; F_zWFL input; F_zWRR input; F_zWRL input; y_FR input; y_FL input; y_RR input; y_RL input; ydot_FR input; ydot_FL input; ydot_RR input; ydot_RL input
function Z = Chassis8(z,m_C,m_WFR,m_WFL,m_WRR,m_WRL,...
    I_Cy,I_CFx,I_CRx,a,b,d_F,e_F,d_R,e_R,k_C,c_C,k_SFR,k_SFL,k_SRR,k_SRL,...
    k_TFR,k_TFL,k_TRR,k_TRL,c_SFR,c_SFL,c_SRR,c_SRL,c_TFR,c_TFL,...
    c_TRR,c_TRL,F_zC,M_y,M_xF,M_xR,F_zWFR,F_zWFL,F_zWRR,F_zWRL,y_FR,...
    y_FL,y_RR,y_RL,ydot_FR,ydot_FL,ydot_RR,ydot_RL)

Z = [z(2);...
    ...
    (1/m_C) * (F_zC...
    + k_SRR * (z(9) - z(1) - b * z(3) + e_R * z(7))...
    + k_SFR * (z(11) - z(1) + a * z(3) + e_F * z(5))...
    + k_SFL * (z(13) - z(1) + a * z(3) - d_F * z(5))...
    + k_SRL * (z(15) - z(1) - b * z(3) - d_R * z(7))...
    + c_SRR * (z(10) - z(2) - b * z(4) + e_R * z(8))...
    + c_SFR * (z(12) - z(2) + a * z(4) + e_F * z(6))...
    + c_SFL * (z(14) - z(2) + a * z(4) - d_F * z(6))...
    + c_SRL * (z(16) - z(2) - b * z(4) - d_R * z(8)));...
    ...
    z(4);...
    ...
    (1/I_Cy) * (M_y...
    + b * k_SRR * (z(9) - z(1) - b * z(3) + e_R * z(7))...
    - a * k_SFR * (z(11) - z(1) + a * z(3) + e_F * z(5))...
    - a * k_SFL * (z(13) - z(1) + a * z(3) - d_F * z(5))...
    + b * k_SRL * (z(15) - z(1) - b * z(3) - d_R * z(7))...
    + b * c_SRR * (z(10) - z(2) - b * z(4) + e_R * z(8))...
    - a * c_SFR * (z(12) - z(2) + a * z(4) + e_F * z(6))...
    - a * c_SFL * (z(14) - z(2) + a * z(4) - d_F * z(6))...
    + b * c_SRL * (z(16) - z(2) - b * z(4) - d_R * z(8)));...
    ...
    z(6);...
    ...
    (1/I_CFx) * (M_xF...
    - e_F * k_SFR * (z(11) - z(1) + a * z(3) + e_F * z(5))...
    + d_F * k_SFL * (z(13) - z(1) + a * z(3) - d_F * z(5))...
    - k_C * (z(5) - z(7))...
    - e_F * c_SFR * (z(12) - z(2) + a * z(4) + e_F * z(6))...
    + d_F * c_SFL * (z(14) - z(2) + a * z(4) - d_F * z(6))...
    - c_C * (z(6) - z(8)));...
    ...
    z(8);...
    ...
    (1/I_CRx) * (M_xR...
    - e_R * k_SRR * (z(9) - z(1) - b * z(3) + e_R * z(7))...
    + d_F * k_SRL * (z(15) - z(1) - b * z(3) - d_R * z(7))...
    + k_C * (z(5) - z(7))...
    - e_R * c_SRR * (z(10) - z(2) - b * z(4) + e_R * z(8))...
    + d_F * c_SRL * (z(16) - z(2) - b * z(4) - d_R * z(8))...
    + c_C * (z(6) - z(8)));...
    ...
    z(10);...
    ...
    (1/m_WRR) * (F_zWRR ...
    + k_TRR * (y_RR - z(9))...
    - k_SRR * (z(9) - z(1) - b * z(3) + e_R * z(7))...
    + c_TRR * (ydot_RR - z(10))...
    - c_SRR * (z(10) - z(2) - b * z(4) + e_R * z(8)));...
    ...
    z(12);...
    ...
    (1/m_WFR) * (F_zWFR ...
    + k_TFR * (y_FR - z(11))...
    - k_SFR * (z(11) - z(1) + a * z(3) + e_F * z(5))...
    + c_TFR * (ydot_FR - z(12))...
    - c_SFR * (z(12) - z(2) + a * z(4) + e_F * z(6)));...
    ...
    z(14);...
    ...
    (1/m_WFL) * (F_zWFL ...
    + k_TFL * (y_FL - z(13))...
    - k_SFL * (z(13) - z(1) + a * z(3) - d_F * z(5))...
    + c_TFL * (ydot_FL - z(14))...
    - c_SFL * (z(14) - z(2) + a * z(4) - d_F * z(6)));...
    ...
    z(16);...
    ...
    (1/m_WRL) * (F_zWRL ...
    + k_TRL * (y_RL - z(15))...
    - k_SRL * (z(15) - z(1) - b * z(3) - d_R * z(7))...
    + c_TRL * (ydot_RL - z(16))...
    - c_SRL * (z(16) - z(2) - b * z(4) - d_R * z(8)))...
    ];

end

== matlab function Vehicle_Model/Subsystem/MATLAB Function18 ==
  data: g input; F_y output; m_C input; h_C input; m_CF input; m_CR input; h_CF input; h_CR input; a input; b input; d_F input; e_F input; d_R input; e_R input; F_yFR input; F_yFL input; F_yRR input; F_yRL input; F_xFR input; F_xFL input; F_xRR input; F_xRL input; M_zFR input; M_zFL input; M_zRR input; M_zRL input; S_FR input; S_FL input; S_RR input; S_RL input; m_WRL input; m_WRR input; m_WFL input; m_WFR input; F_x output; M_z output; M_y output; M_xF output; M_xR output; F_z output
function [F_y,F_x,M_z,M_y,M_xF,M_xR,F_z] = Chassis7(g,m_C,h_C,m_CF,m_CR,...
    h_CF,h_CR,a,b,d_F,e_F,d_R,e_R,F_yFR,F_yFL,F_yRR,F_yRL,F_xFR,F_xFL,...
    F_xRR,F_xRL,M_zFR,M_zFL,M_zRR,M_zRL,S_FR,S_FL,S_RR,S_RL,m_WRL,m_WRR,...
    m_WFL,m_WFR)

F_y = F_yRL * cos(S_RL) + F_yRR * cos(S_RR) + F_yFL * cos(S_FL) + ...
    F_yFR * cos(S_FR)...
     - F_xRL * sin(S_RL) - F_xRR * sin(S_RR) + F_xFL * sin(S_FL) + ...
    F_xFR * sin(S_FR);

F_x = F_xRL * cos(S_RL) + F_xRR * cos(S_RR) + F_xFL * cos(S_FL) + ...
    F_xFR * cos(S_FR)...
     + F_yRL * sin(S_RL) + F_yRR * sin(S_RR) - F_yFL * sin(S_FL) - ...
    F_yFR * sin(S_FR);

F_z = -g * m_C;

M_z = F_xRR * (sin(S_RR) * b + cos(S_RR) * e_R) +...
    F_yRR * (sin(S_RR) * e_R - cos(S_RR) * b) +...
    F_xFR * (cos(S_FR) * e_F + sin(S_FR) * a) +...
    F_yFR * (cos(S_FR) * a - sin(S_FR) * e_F) +...
    F_xFL * (-cos(S_FL) * d_F + sin(S_FL) * a) +...
    F_yFL * (cos(S_FL) * a + sin(S_FL) * d_F) +...
    F_xRL * (-cos(S_RL) * d_R + sin(S_RL) * b) +...
    F_yRL * (-sin(S_RL) * d_R - cos(S_RL) * b) +...
    + M_zFL + M_zRL + M_zRR + M_zFR;

m = m_C + m_WRL + m_WRR + m_WFL + m_WFR;
a_x = F_x / m;
a_y = F_y / m;
M_y = m_C * a_x * h_C;
M_xF = m_CF * a_y * h_CF;
M_xR = m_CR * a_y * h_CR;
